simulink model "ad_des_sim3"  (R2023a)
settings: Solver=ode15s  StartTime=0.0  StopTime=simulation_time  RelTol=1e-3
model workspace (MAT data in the model file):
  adsorpQ = SimulinkDemos.Signal
  adsorpQ.DataType = 'auto'
  adsorpQ.Dimensions = -1
  adsorpQ.DimensionsMode = 'auto'
  adsorpQ.Complexity = 'auto'
  adsorpQ.SampleTime = -1
  adsorpQ.SamplingMode = 'auto'
values from neighbouring files (symbols this model uses):
  Adsorption_time = 145    [run_this_file.m]
  Desorption_time = 55    [run_this_file.m]
  Rinsing_time = 0    [run_this_file.m]
settings Model: Creator=saasa  LastModifiedBy=ASUSTEK
settings SolverCC: AlgebraicLoopSolver=TrustRegion
settings DebuggingCC: UnconnectedInputMsg=warning  UnconnectedOutputMsg=warning  UnconnectedLineMsg=warning
settings ModelReferenceCC: EnableRefExpFcnMdlSchedulingChecks=on

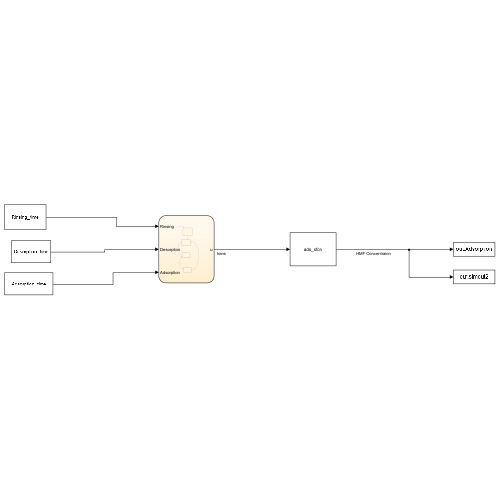
[thumbnail: Simulink's stored preview of the top-level diagram]
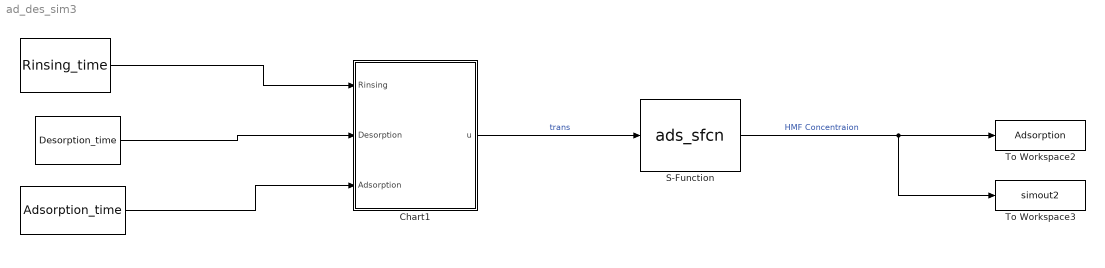
== system ad_des_sim3 ==
  " " : Constant  Value=Rinsing_time
  "  " : Constant  Value=Desorption_time
  "   " : Constant  Value=Adsorption_time
  Chart1 : Stateflow chart  TreatAsAtomicUnit=on
  S-Function : S-Function  FunctionName=ads_sfcn  SFunctionDeploymentMode=off  EnableBusSupport=off
  To Workspace2 : ToWorkspace  VariableName=Adsorption  SampleTime=-1
  To Workspace3 : ToWorkspace  VariableName=simout2  SaveFormat=Timeseries  SampleTime=-1
  wires:
  Chart1/1(u) -> S-Function/1  "trans"
  "  "/1 -> Chart1/2(Desorption)
  "   "/1 -> Chart1/3(Adsorption)
  " "/1 -> Chart1/1(Rinsing)
  S-Function/1 -> To Workspace2/1, To Workspace3/1  "HMF Concentraion"

== stateflow chart ad_des_sim3/Chart1 ==
  state Adsorption_starter
    entry:
    u=1
  state Desorption
    entry:
    u=2
  state Rinsing
    entry:
    u=3;
  state Adsorption
    entry :
    u=1
  (default) -> Adsorption_starter
  Adsorption_starter -> Desorption : [after(Adsorption,sec)]
  Adsorption -> Desorption : [after(Adsorption,sec)]
  Desorption -> Rinsing : [after(Desorption,sec)]
  Rinsing -> Adsorption : [after(Rinsing,sec)]
  data: Rinsing input; u output; Desorption input; Adsorption input
